simulink model "SEN_transformer_completed"  (R2016a)
settings: Solver=ode45  StartTime=0.0  StopTime=1  RelTol=1e-3
undefined symbols (not defined in the file): D11, Delta
libraries: powerlib x45
settings Model: Creator=CPLAB_9  LastModifiedBy=Shahrukh
settings DataIOCC: LimitDataPoints=on  SaveFormat=Array  SignalLoggingSaveFormat=ModelDataLogs
settings OptimizationCC: ExpressionDepthLimit=2147483647
settings DebuggingCC: UnderspecifiedInitializationDetection=Classic  MergeDetectMultiDrivingBlocksExec=none  SolverPrmCheckMsg=warning  FcnCallInpInsideContextMsg=UseLocalSettings  StateNameClashWarn=warning
settings HardwareCC: ProdBitPerPointer=32  ProdLargestAtomicFloat=None  ProdIntDivRoundTo=Undefined  ProdEndianess=Unspecified  ProdWordSize=32  ProdHWDeviceType=32-bit Generic
settings ModelReferenceCC: PropagateSignalLabelsOutOfModel=off
settings GRTTargetCC: CombineOutputUpdateFcns=off  GRTInterface=on
settings ConfigComp: CovModelRefEnable=Off

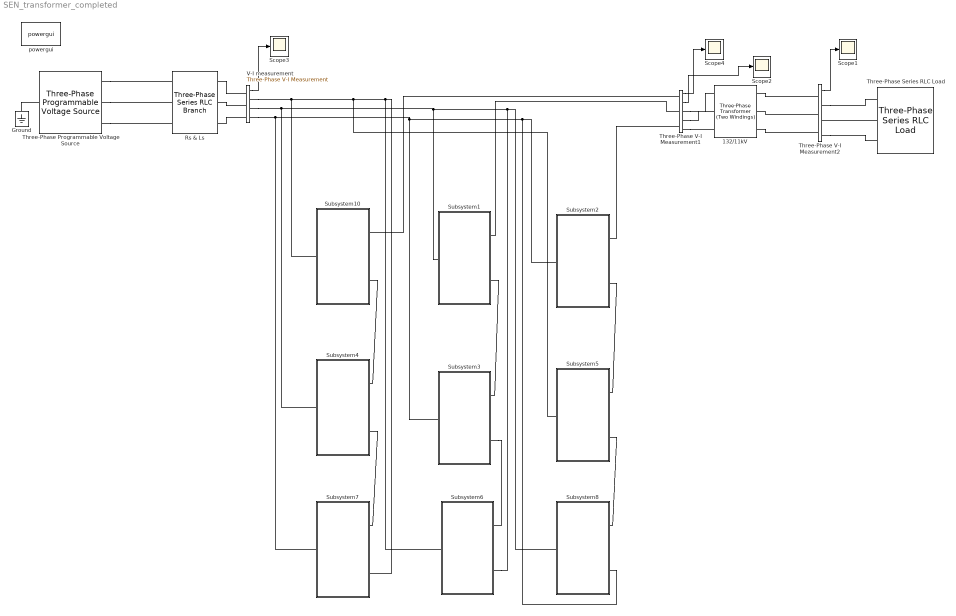
== system SEN_transformer_completed ==
  132/11kV : powerlib/Elements/Three-Phase Transformer (Two Windings)  Winding1Connection=Delta (D11)  Winding2Connection=Delta (D11)  CoreType=Three single-phase transformers  SetSaturation=off  Hysteresis=off  DataFile='hysteresis'  SetInitialFlux=off  Measurements=None  UNITS=pu  NominalPower=[ 132e3 , 50 ]  Winding1="[ 132e3  , 0.1, 0.8 ]"  Winding2=[ 11e3 , 0.01, 0.08 ]  Rm=500  Lm=500  L0=0.5  Saturation=[ 0,0 ; 0.0024,1.2 ; 1.0,1.52 ]  InitialFluxes=[ 0.8 , -0.8 , 0.7 ]  MoreParameters=off  BreakLoop=off  DataType=off  TransfoNumber=1
  Ground : powerlib/Elements/Ground  LConnTagsString=a
  Rs & Ls : powerlib/Elements/Three-Phase Series RLC Branch  LConnTagsString=A|B|C  RConnTagsString=A|B|C  BranchType=RL  Resistance=0.02  Inductance=0.01  Capacitance=1.0  Measurements=Branch voltages
  Scope{1..4} (4 alike) : Scope
  Subsystem1 : Subsystem
  Subsystem10 : Subsystem
  Subsystem2 : Subsystem
  Subsystem3 : Subsystem
  Subsystem4 : Subsystem
  Subsystem5 : Subsystem
  Subsystem6 : Subsystem
  Subsystem7 : Subsystem
  Subsystem8 : Subsystem
  Three-Phase Programmable Voltage Source : powerlib/Electrical Sources/Three-Phase Programmable Voltage Source  PositiveSequence="[132e3  0 50]"  VariationEntity=Amplitude  VariationType=Table of time-amplitude pairs  VariationTypeAlt=Step  VariationStep=0.5  VariationRate=10  VariationMagnitude=0.3  VariationFrequency=2  VariationTiming=[1 2]  VariationPhaseA=off  Amplitudes=[1 1.2 1 1]  TimeValues=[0 0.1 0.4 0.5]  HarmonicGeneration=off  HarmonicA=[3 0.2 -25 0]  HarmonicB=[2 0.15 35 2]  Timing="[0.05  3]"  BusType=swing  Pref=0  Qref=0  Qmin=-inf  Qmax=inf
  Three-Phase Series RLC Load : powerlib/Elements/Three-Phase Series RLC Load  LConnTagsString=A|B|C  Configuration=Y (grounded)  NominalVoltage=11e3  Vabc=[1e3 1e3 1e3]  Vabcp=[1e3 1e3 1e3]  NominalFrequency=50  UnbalancedPower=off  ActivePower=100e3  InductivePower=1000  CapacitivePower=1000  Pabc=[10e3 9e3 11e3]  QLabc=[100 90 110]  QCabc=[100 90 110]  Pabcp=[10e3 9e3 11e3]  QLabcp=[100 90 110]  QCabcp=[100 90 110]  Measurements=Branch voltages  LoadType=constant Z
  Three-Phase V-I Measurement1 : powerlib/Measurements/Three-Phase V-I Measurement  VoltageMeasurement=phase-to-ground  SetLabelV=off  LabelV=Vabc  Vpu=on  VpuLL=off  CurrentMeasurement=yes  SetLabelI=off  LabelI=Iabc  Ipu=off  Pbase=100e6  Vbase=132e3  OutputType=Complex  PhasorSimulation=off  PSBequivalent=0
  Three-Phase V-I Measurement2 : powerlib/Measurements/Three-Phase V-I Measurement  VoltageMeasurement=phase-to-phase  SetLabelV=off  LabelV=Vabc  Vpu=off  VpuLL=on  CurrentMeasurement=no  SetLabelI=off  LabelI=Iabc  Ipu=off  Pbase=100e6  Vbase=11e3  OutputType=Complex  PhasorSimulation=off  PSBequivalent=0
  V-I measurement : powerlib/Measurements/Three-Phase V-I Measurement  VoltageMeasurement=phase-to-ground  SetLabelV=off  LabelV=Vabc  Vpu=on  VpuLL=off  CurrentMeasurement=no  SetLabelI=off  LabelI=Iabc  Ipu=off  Pbase=100e6  Vbase=132e3  OutputType=Complex  PhasorSimulation=off  PSBequivalent=0
  powergui : powerlib/powergui  Priority=1  SimulationMode=Discrete  SolverType=Tustin/Backward Euler (TBE)  SampleTime=50e-6  frequency=60  SPID=off  DisableSnubberDevices=off  DisableRonSwitches=off  DisableVfSwitches=off  SwTol=0  DisplayEquations=off  Interpol=off  ExternalGateDelay=off  methode=off  Ts=10  FunctionMessages=off  echomessages=off  HookPort=off  EnableUseOfTLC=off  x0status=blocks  frequencyindice=50  Pbase=100e6  ErrMax=1e-4  Iterations=50  UnitsV=kV  UnitsW=MW  buscounter=0  RestoreLinks=warning  ResistiveCurrentMeasurement=off  Frange=[0:2:500]  Ylog=off  Xlog=on  ShowGrid=off  save=off  variable=ZData  structure=0  ZoomFFT=off  StartTime=0.0  cycles=1  DisplayStyle=1  fundamental=60  FreqAxis=off  MaxFrequency=1000  frequencyindicesteady=1  RmsSteady=1  display=off
  wires:
  V-I measurement/1 -> Scope3/1
  Three-Phase V-I Measurement1/1 -> Scope4/1
  Three-Phase V-I Measurement2/1 -> Scope1/1
  Three-Phase V-I Measurement1/2 -> Scope2/1
  connections:
  Three-Phase Programmable Voltage Source/RConn1 -- Rs & Ls/LConn1
  Three-Phase Programmable Voltage Source/RConn2 -- Rs & Ls/LConn2
  Three-Phase Programmable Voltage Source/RConn3 -- Rs & Ls/LConn3
  Rs & Ls/RConn1 -- V-I measurement/LConn1
  Rs & Ls/RConn2 -- V-I measurement/LConn2
  Rs & Ls/RConn3 -- V-I measurement/LConn3
  Ground/LConn1 -- Three-Phase Programmable Voltage Source/LConn1
  Three-Phase V-I Measurement1/RConn1 -- 132/11kV/LConn1
  Three-Phase V-I Measurement1/RConn2 -- 132/11kV/LConn2
  Three-Phase V-I Measurement1/RConn3 -- 132/11kV/LConn3
  Three-Phase Series RLC Load/LConn2 -- Three-Phase V-I Measurement2/RConn2
  132/11kV/RConn3 -- Three-Phase V-I Measurement2/LConn3
  Three-Phase V-I Measurement2/LConn2 -- 132/11kV/RConn2
  132/11kV/RConn1 -- Three-Phase V-I Measurement2/LConn1
  Three-Phase V-I Measurement2/RConn3 -- Three-Phase Series RLC Load/LConn3
  Three-Phase V-I Measurement2/RConn1 -- Three-Phase Series RLC Load/LConn1
  Subsystem10/LConn2 -- Subsystem4/LConn1
  Subsystem4/LConn2 -- Subsystem7/LConn1
  V-I measurement/RConn1 -- Subsystem10/RConn1 -- Subsystem5/RConn1 -- Subsystem6/RConn1 -- Subsystem7/LConn2
  Three-Phase V-I Measurement1/LConn1 -- Subsystem10/LConn1
  Three-Phase V-I Measurement1/LConn2 -- Subsystem1/LConn1
  Subsystem1/LConn2 -- Subsystem3/LConn1
  V-I measurement/RConn2 -- Subsystem4/RConn1 -- Subsystem6/LConn2 -- Subsystem8/RConn1 -- Subsystem1/RConn1
  V-I measurement/RConn3 -- Subsystem7/RConn1 -- Subsystem8/LConn2 -- Subsystem2/RConn1 -- Subsystem3/RConn1
  Subsystem3/LConn2 -- Subsystem6/LConn1
  Three-Phase V-I Measurement1/LConn3 -- Subsystem2/LConn1
  Subsystem2/LConn2 -- Subsystem5/LConn1
  Subsystem5/LConn2 -- Subsystem8/LConn1

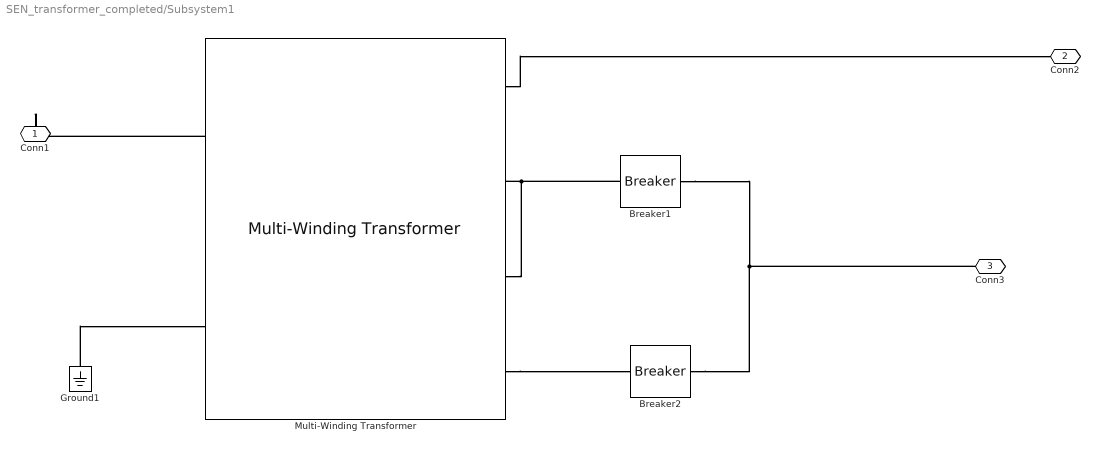
== system SEN_transformer_completed/Subsystem1 ==
  Breaker1 : powerlib/Elements/Breaker  InitialState=0  SwitchingTimes=[0 1]  External=off  BreakerResistance=0.01  SnubberResistance=1e6  SnubberCapacitance=inf  Measurements=None  MoreParameters=on  NoBreakLoop=off
  Breaker2 : powerlib/Elements/Breaker  InitialState=1  SwitchingTimes=[0 1]  External=off  BreakerResistance=0.01  SnubberResistance=1e6  SnubberCapacitance=inf  Measurements=None  MoreParameters=on  NoBreakLoop=off
  Ground1 : powerlib/Elements/Ground  LConnTagsString=a
  Multi-Winding Transformer : powerlib/Elements/Multi-Winding Transformer  LeftWindings=1  RightWindings=2  TappedWindings=no taps  NumberOfTaps=2  UNITS=pu  NominalPower=[132e3 50]  NominalVoltages=[ 76210 3810.5 12500 ]  WindingResistances="[ 0.005  0.005  0.005  0.005]"  WindingInductances="[ 0.02  0.02  0.02  0.02 ]"  SetSaturation=off  Rm=50  Lm=50  Saturation=[ 0,0 ; 0.0024,1.2 ; 1.0,1.52 ]  Hysteresis=off  DataFile='hysteresis.mat'  Measurements=None  MoreParameters=off  BreakLoop=off  DataType=off  InitialFlux=0  TransfoNumber=1
  Conn1 : PMIOPort  Port=1  Side=Right
  Conn2 : PMIOPort  Port=2  Side=Left
  Conn3 : PMIOPort  Port=3  Side=Left
  connections:
  Breaker1/RConn1 -- Breaker2/RConn1 -- Conn3/RConn1
  Ground1/LConn1 -- Multi-Winding Transformer/LConn2
  Breaker1/LConn1 -- Multi-Winding Transformer/RConn3 -- Multi-Winding Transformer/RConn2
  Multi-Winding Transformer/RConn1 -- Conn2/RConn1
  Multi-Winding Transformer/LConn1 -- Conn1/RConn1
  Multi-Winding Transformer/RConn4 -- Breaker2/LConn1

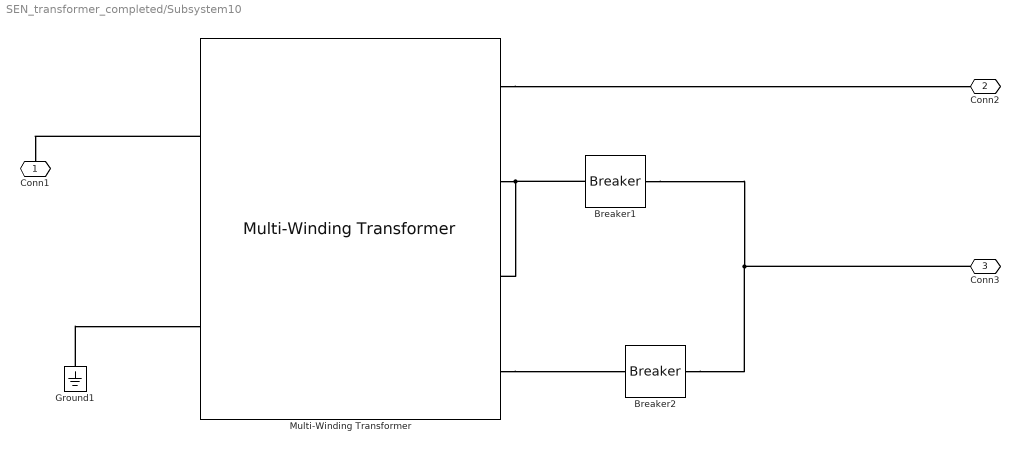
== system SEN_transformer_completed/Subsystem10 ==
  Breaker1 : powerlib/Elements/Breaker  InitialState=0  SwitchingTimes=[0 1]  External=off  BreakerResistance=0.0001  SnubberResistance=1e6  SnubberCapacitance=inf  Measurements=None  MoreParameters=on  NoBreakLoop=off
  Breaker2 : powerlib/Elements/Breaker  InitialState=1  SwitchingTimes=[0 1]  External=off  BreakerResistance=0.01  SnubberResistance=1e6  SnubberCapacitance=inf  Measurements=None  MoreParameters=on  NoBreakLoop=off
  Ground1 : powerlib/Elements/Ground  LConnTagsString=a
  Multi-Winding Transformer : powerlib/Elements/Multi-Winding Transformer  LeftWindings=1  RightWindings=2  TappedWindings=no taps  NumberOfTaps=2  UNITS=pu  NominalPower=[50e3 50]  NominalVoltages=[ 76210 3810.5 12500 ]  WindingResistances="[ 0.0005  0.0005  0.0005  0.0005]"  WindingInductances="[ 0.002  0.002  0.002  0.002 ]"  SetSaturation=off  Rm=500  Lm=500  Saturation=[ 0,0 ; 0.0024,1.2 ; 1.0,1.52 ]  Hysteresis=off  DataFile='hysteresis.mat'  Measurements=None  MoreParameters=off  BreakLoop=off  DataType=off  InitialFlux=0  TransfoNumber=1
  Conn1 : PMIOPort  Port=1  Side=Right
  Conn2 : PMIOPort  Port=2  Side=Left
  Conn3 : PMIOPort  Port=3  Side=Left
  connections:
  Breaker1/RConn1 -- Breaker2/RConn1 -- Conn3/RConn1
  Ground1/LConn1 -- Multi-Winding Transformer/LConn2
  Multi-Winding Transformer/RConn1 -- Conn2/RConn1
  Multi-Winding Transformer/LConn1 -- Conn1/RConn1
  Multi-Winding Transformer/RConn4 -- Breaker2/LConn1
  Multi-Winding Transformer/RConn2 -- Breaker1/LConn1 -- Multi-Winding Transformer/RConn3

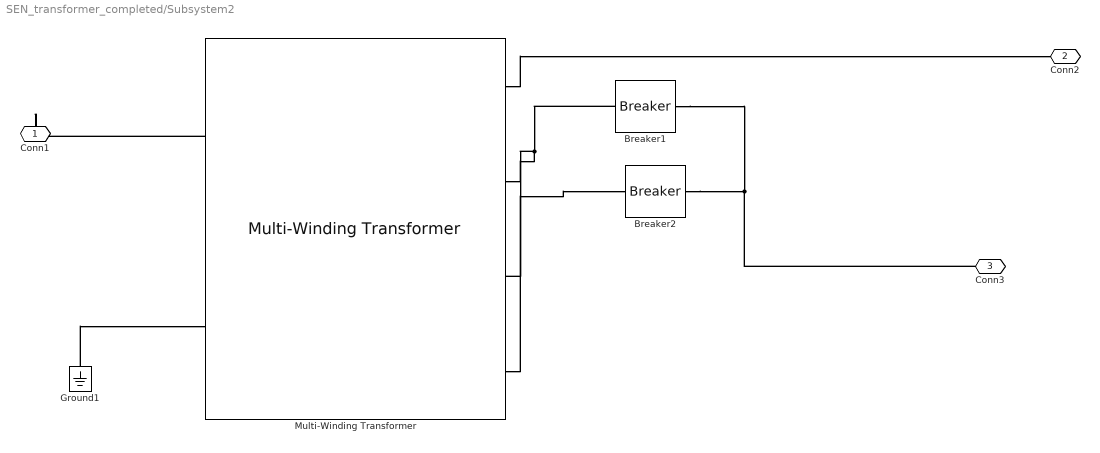
== system SEN_transformer_completed/Subsystem2 ==
  Breaker1 : powerlib/Elements/Breaker  InitialState=0  SwitchingTimes=[0 1]  External=off  BreakerResistance=0.01  SnubberResistance=1e6  SnubberCapacitance=inf  Measurements=None  MoreParameters=on  NoBreakLoop=off
  Breaker2 : powerlib/Elements/Breaker  InitialState=1  SwitchingTimes=[0 1]  External=off  BreakerResistance=0.01  SnubberResistance=1e6  SnubberCapacitance=inf  Measurements=None  MoreParameters=on  NoBreakLoop=off
  Ground1 : powerlib/Elements/Ground  LConnTagsString=a
  Multi-Winding Transformer : powerlib/Elements/Multi-Winding Transformer  LeftWindings=1  RightWindings=2  TappedWindings=no taps  NumberOfTaps=2  UNITS=pu  NominalPower=[132e3 50]  NominalVoltages=[ 76210 3810.5 12500 ]  WindingResistances="[ 0.005  0.005  0.005  0.005]"  WindingInductances="[ 0.02  0.02  0.02  0.02 ]"  SetSaturation=off  Rm=50  Lm=50  Saturation=[ 0,0 ; 0.0024,1.2 ; 1.0,1.52 ]  Hysteresis=off  DataFile='hysteresis.mat'  Measurements=None  MoreParameters=off  BreakLoop=off  DataType=off  InitialFlux=0  TransfoNumber=1
  Conn1 : PMIOPort  Port=1  Side=Right
  Conn2 : PMIOPort  Port=2  Side=Left
  Conn3 : PMIOPort  Port=3  Side=Left
  connections:
  Breaker1/RConn1 -- Conn3/RConn1 -- Breaker2/RConn1
  Ground1/LConn1 -- Multi-Winding Transformer/LConn2
  Multi-Winding Transformer/RConn2 -- Multi-Winding Transformer/RConn3 -- Breaker1/LConn1
  Multi-Winding Transformer/RConn1 -- Conn2/RConn1
  Multi-Winding Transformer/LConn1 -- Conn1/RConn1
  Multi-Winding Transformer/RConn4 -- Breaker2/LConn1

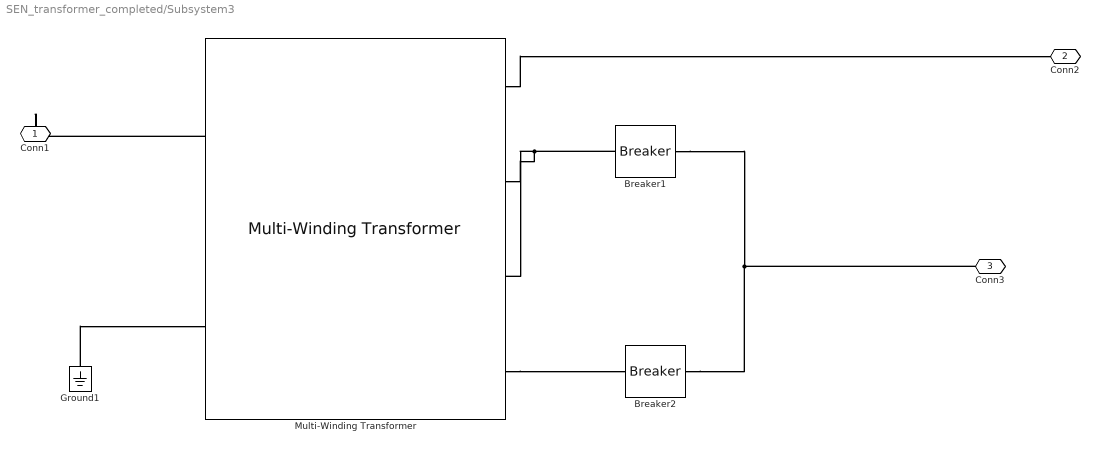
== system SEN_transformer_completed/Subsystem3 ==
  Breaker1 : powerlib/Elements/Breaker  InitialState=1  SwitchingTimes=[0.1 0.4]  External=off  BreakerResistance=0.01  SnubberResistance=1e6  SnubberCapacitance=inf  Measurements=None  MoreParameters=on  NoBreakLoop=off
  Breaker2 : powerlib/Elements/Breaker  InitialState=0  SwitchingTimes=[0.1 0.4]  External=off  BreakerResistance=0.01  SnubberResistance=1e6  SnubberCapacitance=inf  Measurements=None  MoreParameters=on  NoBreakLoop=off
  Ground1 : powerlib/Elements/Ground  LConnTagsString=a
  Multi-Winding Transformer : powerlib/Elements/Multi-Winding Transformer  LeftWindings=1  RightWindings=2  TappedWindings=no taps  NumberOfTaps=2  UNITS=pu  NominalPower=[132e3 50]  NominalVoltages=[ 76210 3810.5 12500 ]  WindingResistances="[ 0.005  0.005  0.005  0.005]"  WindingInductances="[ 0.02  0.02  0.02  0.02 ]"  SetSaturation=off  Rm=50  Lm=50  Saturation=[ 0,0 ; 0.0024,1.2 ; 1.0,1.52 ]  Hysteresis=off  DataFile='hysteresis.mat'  Measurements=None  MoreParameters=off  BreakLoop=off  DataType=off  InitialFlux=0  TransfoNumber=1
  Conn1 : PMIOPort  Port=1  Side=Right
  Conn2 : PMIOPort  Port=2  Side=Left
  Conn3 : PMIOPort  Port=3  Side=Left
  connections:
  Breaker1/RConn1 -- Breaker2/RConn1 -- Conn3/RConn1
  Ground1/LConn1 -- Multi-Winding Transformer/LConn2
  Multi-Winding Transformer/RConn2 -- Breaker1/LConn1 -- Multi-Winding Transformer/RConn3
  Multi-Winding Transformer/RConn1 -- Conn2/RConn1
  Multi-Winding Transformer/LConn1 -- Conn1/RConn1
  Multi-Winding Transformer/RConn4 -- Breaker2/LConn1

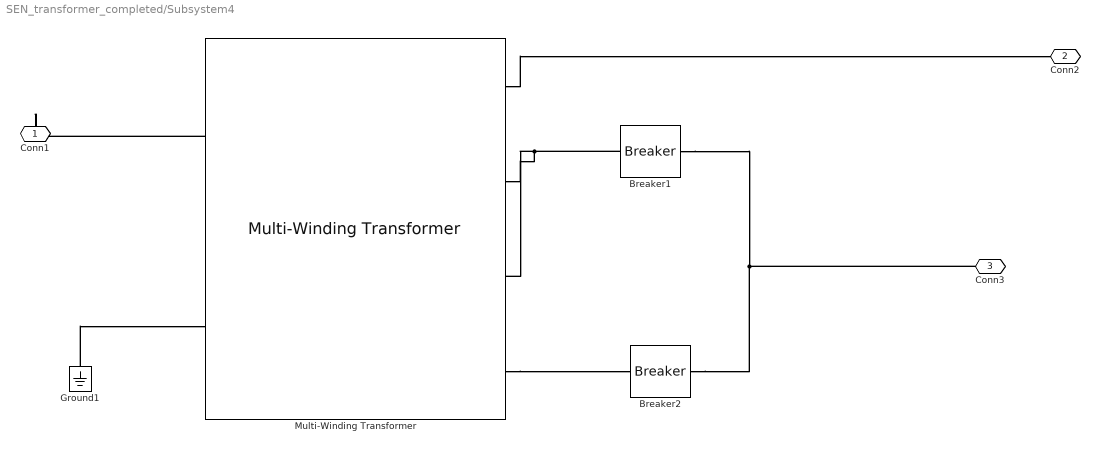
== system SEN_transformer_completed/Subsystem4 ==
  Breaker1 : powerlib/Elements/Breaker  InitialState=1  SwitchingTimes=[0.1 0.4]  External=off  BreakerResistance=0.0001  SnubberResistance=1e6  SnubberCapacitance=inf  Measurements=None  MoreParameters=on  NoBreakLoop=off
  Breaker2 : powerlib/Elements/Breaker  InitialState=0  SwitchingTimes=[0.1 0.4]  External=off  BreakerResistance=0.0001  SnubberResistance=1e6  SnubberCapacitance=inf  Measurements=None  MoreParameters=on  NoBreakLoop=off
  Ground1 : powerlib/Elements/Ground  LConnTagsString=a
  Multi-Winding Transformer : powerlib/Elements/Multi-Winding Transformer  LeftWindings=1  RightWindings=2  TappedWindings=no taps  NumberOfTaps=2  UNITS=pu  NominalPower=[50e3 50]  NominalVoltages=[ 76210 3810.5 12500 ]  WindingResistances="[ 0.0005  0.0005  0.0005  0.0005]"  WindingInductances="[ 0.002  0.002  0.002  0.0002 ]"  SetSaturation=off  Rm=500  Lm=500  Saturation=[ 0,0 ; 0.0024,1.2 ; 1.0,1.52 ]  Hysteresis=off  DataFile='hysteresis.mat'  Measurements=None  MoreParameters=off  BreakLoop=off  DataType=off  InitialFlux=0  TransfoNumber=1
  Conn1 : PMIOPort  Port=1  Side=Right
  Conn2 : PMIOPort  Port=2  Side=Left
  Conn3 : PMIOPort  Port=3  Side=Left
  connections:
  Breaker1/RConn1 -- Breaker2/RConn1 -- Conn3/RConn1
  Ground1/LConn1 -- Multi-Winding Transformer/LConn2
  Multi-Winding Transformer/RConn2 -- Breaker1/LConn1 -- Multi-Winding Transformer/RConn3
  Multi-Winding Transformer/RConn1 -- Conn2/RConn1
  Multi-Winding Transformer/LConn1 -- Conn1/RConn1
  Multi-Winding Transformer/RConn4 -- Breaker2/LConn1

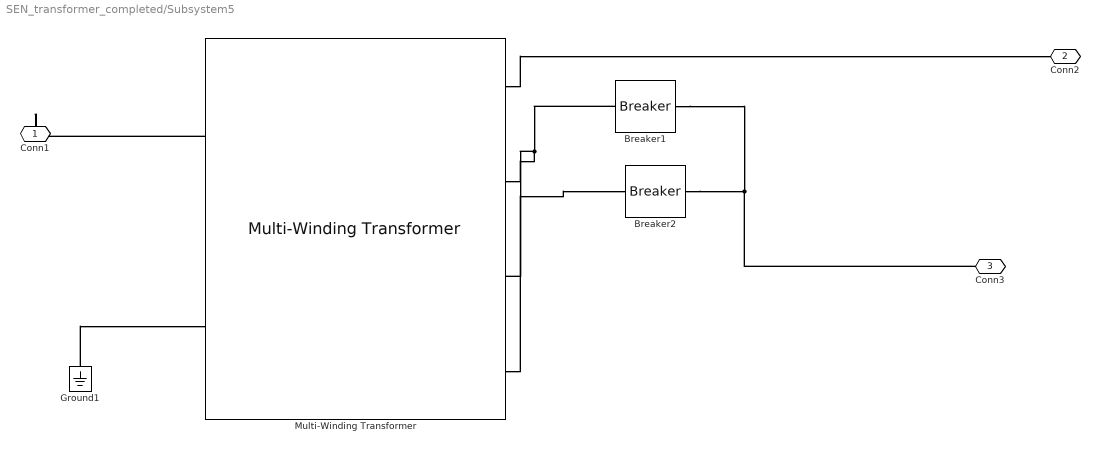
== system SEN_transformer_completed/Subsystem5 ==
  Breaker1 : powerlib/Elements/Breaker  InitialState=1  SwitchingTimes=[0.1 0.4]  External=off  BreakerResistance=0.01  SnubberResistance=1e6  SnubberCapacitance=inf  Measurements=None  MoreParameters=on  NoBreakLoop=off
  Breaker2 : powerlib/Elements/Breaker  InitialState=0  SwitchingTimes=[0.1 0.4]  External=off  BreakerResistance=0.01  SnubberResistance=1e6  SnubberCapacitance=inf  Measurements=None  MoreParameters=on  NoBreakLoop=off
  Ground1 : powerlib/Elements/Ground  LConnTagsString=a
  Multi-Winding Transformer : powerlib/Elements/Multi-Winding Transformer  LeftWindings=1  RightWindings=2  TappedWindings=no taps  NumberOfTaps=2  UNITS=pu  NominalPower=[132e3 50]  NominalVoltages=[ 76210 3810.5 12500 ]  WindingResistances="[ 0.005  0.005  0.005  0.005]"  WindingInductances="[ 0.02  0.02  0.02  0.02 ]"  SetSaturation=off  Rm=50  Lm=50  Saturation=[ 0,0 ; 0.0024,1.2 ; 1.0,1.52 ]  Hysteresis=off  DataFile='hysteresis.mat'  Measurements=None  MoreParameters=off  BreakLoop=off  DataType=off  InitialFlux=0  TransfoNumber=1
  Conn1 : PMIOPort  Port=1  Side=Right
  Conn2 : PMIOPort  Port=2  Side=Left
  Conn3 : PMIOPort  Port=3  Side=Left
  connections:
  Breaker1/RConn1 -- Conn3/RConn1 -- Breaker2/RConn1
  Ground1/LConn1 -- Multi-Winding Transformer/LConn2
  Multi-Winding Transformer/RConn2 -- Multi-Winding Transformer/RConn3 -- Breaker1/LConn1
  Multi-Winding Transformer/RConn1 -- Conn2/RConn1
  Multi-Winding Transformer/LConn1 -- Conn1/RConn1
  Multi-Winding Transformer/RConn4 -- Breaker2/LConn1

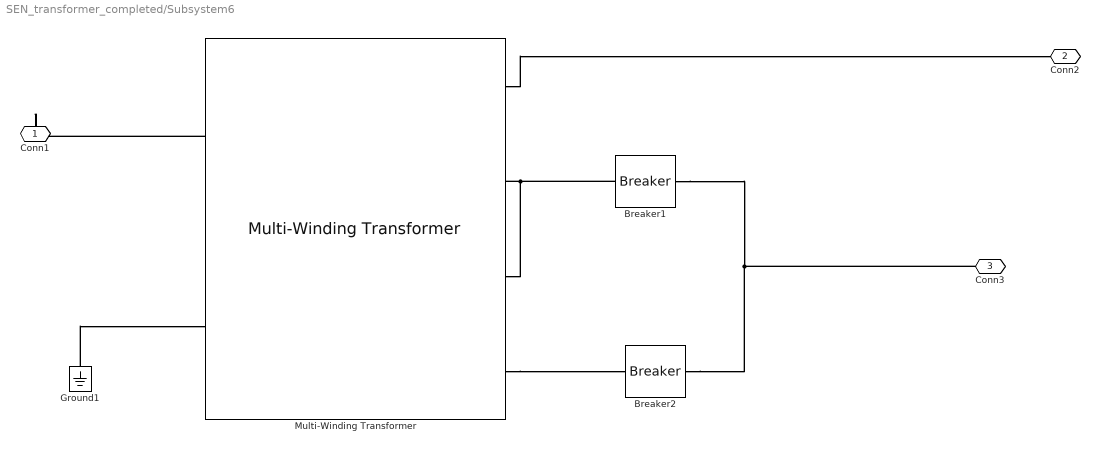
== system SEN_transformer_completed/Subsystem6 ==
  Breaker1 : powerlib/Elements/Breaker  InitialState=1  SwitchingTimes=[0.1 0.4]  External=off  BreakerResistance=0.01  SnubberResistance=1e6  SnubberCapacitance=inf  Measurements=None  MoreParameters=on  NoBreakLoop=off
  Breaker2 : powerlib/Elements/Breaker  InitialState=0  SwitchingTimes=[0.1 0.4]  External=off  BreakerResistance=0.01  SnubberResistance=1e6  SnubberCapacitance=inf  Measurements=None  MoreParameters=on  NoBreakLoop=off
  Ground1 : powerlib/Elements/Ground  LConnTagsString=a
  Multi-Winding Transformer : powerlib/Elements/Multi-Winding Transformer  LeftWindings=1  RightWindings=2  TappedWindings=no taps  NumberOfTaps=2  UNITS=pu  NominalPower=[132e3 50]  NominalVoltages=[ 76210 3810.5 12500 ]  WindingResistances="[ 0.005  0.005  0.005  0.005]"  WindingInductances="[ 0.02  0.02  0.02  0.02 ]"  SetSaturation=off  Rm=50  Lm=50  Saturation=[ 0,0 ; 0.0024,1.2 ; 1.0,1.52 ]  Hysteresis=off  DataFile='hysteresis.mat'  Measurements=None  MoreParameters=off  BreakLoop=off  DataType=off  InitialFlux=0  TransfoNumber=1
  Conn1 : PMIOPort  Port=1  Side=Right
  Conn2 : PMIOPort  Port=2  Side=Left
  Conn3 : PMIOPort  Port=3  Side=Left
  connections:
  Breaker1/RConn1 -- Conn3/RConn1 -- Breaker2/RConn1
  Ground1/LConn1 -- Multi-Winding Transformer/LConn2
  Multi-Winding Transformer/RConn1 -- Conn2/RConn1
  Multi-Winding Transformer/LConn1 -- Conn1/RConn1
  Multi-Winding Transformer/RConn4 -- Breaker2/LConn1
  Multi-Winding Transformer/RConn3 -- Breaker1/LConn1 -- Multi-Winding Transformer/RConn2

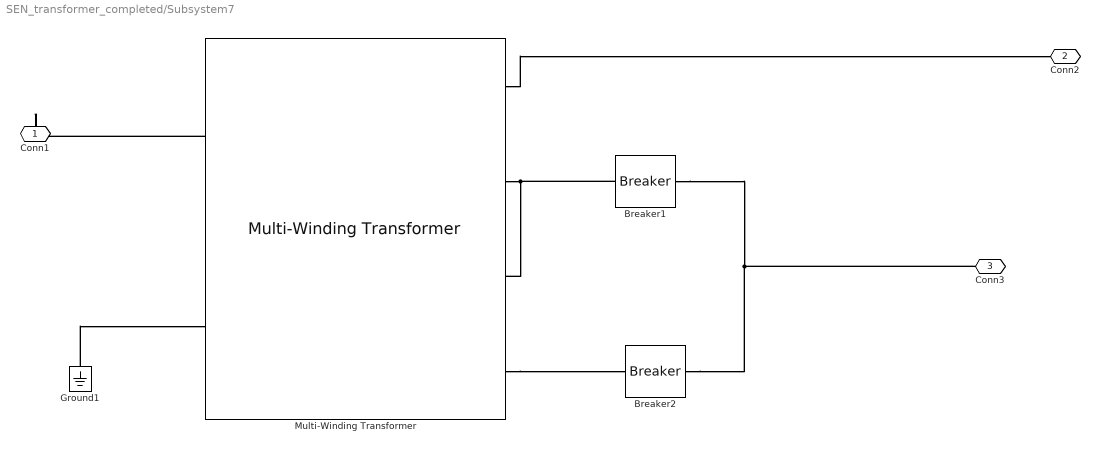
== system SEN_transformer_completed/Subsystem7 ==
  Breaker1 : powerlib/Elements/Breaker  InitialState=1  SwitchingTimes=[0.1 0.4]  External=off  BreakerResistance=0.0001  SnubberResistance=1e6  SnubberCapacitance=inf  Measurements=None  MoreParameters=on  NoBreakLoop=off
  Breaker2 : powerlib/Elements/Breaker  InitialState=0  SwitchingTimes=[0.1 0.4]  External=off  BreakerResistance=0.0001  SnubberResistance=1e6  SnubberCapacitance=inf  Measurements=None  MoreParameters=on  NoBreakLoop=off
  Ground1 : powerlib/Elements/Ground  LConnTagsString=a
  Multi-Winding Transformer : powerlib/Elements/Multi-Winding Transformer  LeftWindings=1  RightWindings=2  TappedWindings=no taps  NumberOfTaps=2  UNITS=pu  NominalPower=[50e3 50]  NominalVoltages=[ 76210 3810.5 12500 ]  WindingResistances="[ 0.0005  0.0005  0.0005  0.0005]"  WindingInductances="[ 0.002  0.002  0.002  0.002 ]"  SetSaturation=off  Rm=500  Lm=500  Saturation=[ 0,0 ; 0.0024,1.2 ; 1.0,1.52 ]  Hysteresis=off  DataFile='hysteresis.mat'  Measurements=None  MoreParameters=off  BreakLoop=off  DataType=off  InitialFlux=0  TransfoNumber=1
  Conn1 : PMIOPort  Port=1  Side=Right
  Conn2 : PMIOPort  Port=2  Side=Left
  Conn3 : PMIOPort  Port=3  Side=Left
  connections:
  Breaker1/RConn1 -- Conn3/RConn1 -- Breaker2/RConn1
  Ground1/LConn1 -- Multi-Winding Transformer/LConn2
  Breaker1/LConn1 -- Multi-Winding Transformer/RConn2 -- Multi-Winding Transformer/RConn3
  Multi-Winding Transformer/RConn1 -- Conn2/RConn1
  Multi-Winding Transformer/LConn1 -- Conn1/RConn1
  Multi-Winding Transformer/RConn4 -- Breaker2/LConn1

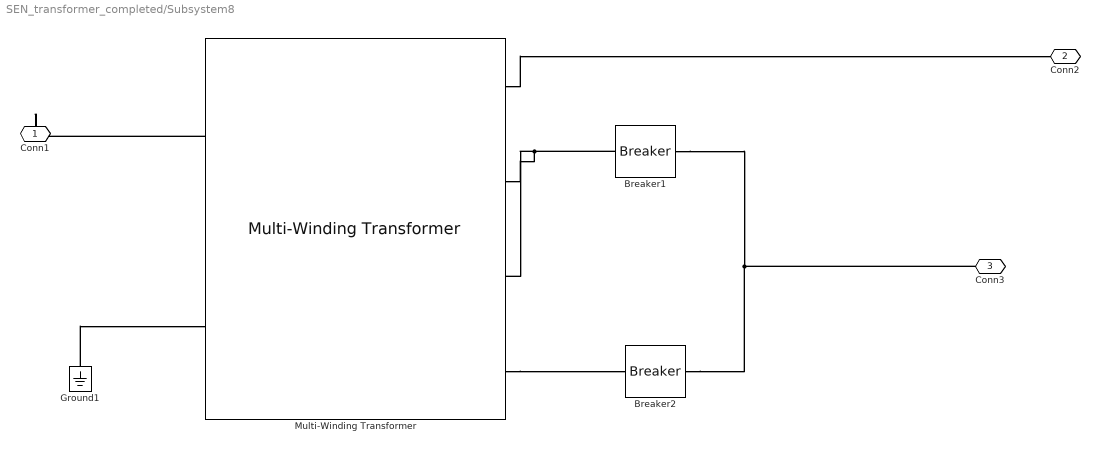
== system SEN_transformer_completed/Subsystem8 ==
  Breaker1 : powerlib/Elements/Breaker  InitialState=1  SwitchingTimes=[0.1 0.4]  External=off  BreakerResistance=0.01  SnubberResistance=1e6  SnubberCapacitance=inf  Measurements=None  MoreParameters=on  NoBreakLoop=off
  Breaker2 : powerlib/Elements/Breaker  InitialState=0  SwitchingTimes=[0.1 0.4]  External=off  BreakerResistance=0.01  SnubberResistance=1e6  SnubberCapacitance=inf  Measurements=None  MoreParameters=on  NoBreakLoop=off
  Ground1 : powerlib/Elements/Ground  LConnTagsString=a
  Multi-Winding Transformer : powerlib/Elements/Multi-Winding Transformer  LeftWindings=1  RightWindings=2  TappedWindings=no taps  NumberOfTaps=2  UNITS=pu  NominalPower=[132e3 50]  NominalVoltages=[ 76210 3810.5 12500 ]  WindingResistances="[ 0.005  0.005  0.005  0.005]"  WindingInductances="[ 0.02  0.02  0.02  0.02 ]"  SetSaturation=off  Rm=50  Lm=50  Saturation=[ 0,0 ; 0.0024,1.2 ; 1.0,1.52 ]  Hysteresis=off  DataFile='hysteresis.mat'  Measurements=None  MoreParameters=off  BreakLoop=off  DataType=off  InitialFlux=0  TransfoNumber=1
  Conn1 : PMIOPort  Port=1  Side=Right
  Conn2 : PMIOPort  Port=2  Side=Left
  Conn3 : PMIOPort  Port=3  Side=Left
  connections:
  Breaker1/RConn1 -- Breaker2/RConn1 -- Conn3/RConn1
  Ground1/LConn1 -- Multi-Winding Transformer/LConn2
  Multi-Winding Transformer/RConn2 -- Breaker1/LConn1 -- Multi-Winding Transformer/RConn3
  Multi-Winding Transformer/RConn1 -- Conn2/RConn1
  Multi-Winding Transformer/LConn1 -- Conn1/RConn1
  Multi-Winding Transformer/RConn4 -- Breaker2/LConn1
